simulink model "sf_electrohydraulic"  (Simulink 7.6)
settings: Solver=ode45  SolverMode=SingleTasking  StartTime=0.0  StopTime=2  FixedStep=0.2e-4  RelTol=1e-6
model workspace (MAT data in the model file):
  BHcurve.H = [-11439.2615347; -7246.13776302; -3771.53605391; -987.067511384; -118.29393547; -78.4550283852; -44.7231237731; -17.3583519401; -13.039382708; -10.5700097302; -8.52378165855; -6.82818955541; -5.42314941344; -4.25887305422; -3.43177169131; -2.84371281009; -2.35642206816; -1.95263211657; -1.61803449144; -1.34077258756; -1.11102151473; -0.920639948664; -0.762881639861; -0.632156357415; -0.523831796886; -0.434069432681; -0.359688498308; -0.298053274602; -0.246979691925; -0.204657936755; -0.1695883202; -0.140528135894; -0.116447624191; -0.0964934822022; -0.0799586266544; -0.0662571381046; -0.0549034986404; -0.0454953873528; -0.0376994239281; -0.0312393551788; -0.0258862658976; -0.0214504671522; -0.01777477458; -0.0147289384949; -0.0122050284356; -0.0101136086056; -0.00838056867855; -0.00694449766789; -0.0057545078036; -0.00476843130279; 0; 0.00476843130279; 0.0057545078036; 0.00694449766789; 0.00838056867855; 0.0101136086056; 0.0122050284356; 0.0147289384949; 0.01777477458; 0.0214504671522; 0.0258862658976; 0.0312393551788; 0.0376994239281; 0.0454953873528; 0.0549034986404; 0.0662571381046; 0.0799586266544; 0.0964934822022; 0.116447624191; 0.140528135894; 0.1695883202; 0.204657936755; 0.246979691925; 0.298053274602; 0.359688498308; 0.434069432681; 0.523831796886; 0.632156357415; 0.762881639861; 0.920639948664; 1.11102151473; 1.34077258756; 1.61803449144; 1.95263211657; 2.35642206816; 2.84371281009; 3.43177169131; 4.25887305422; 5.42314941344; 6.82818955541; 8.52378165855; 10.5700097302; 13.039382708; 16.3583519401; 43.7231237731; 77.4550283852; 118.29393547; 987.067511384; 3771.53605391; 7246.13776302; 11439.2615347]
  BHcurve.B = [-3; -2.48592831856; -2.05994653501; -1.70695980871; -1.41445990904; -1.17208198112; -0.971237262845; -0.804808738584; -0.666898944758; -0.552620990798; -0.457925390153; -0.379456565057; -0.314433940246; -0.260553412125; -0.2159057019; -0.178908699498; -0.14825140084; -0.122847451871; -0.101796653157; -0.0843530609392; -0.0698985543155; -0.0579209318665; -0.0479957615882; -0.0397713409677; -0.0329562342596; -0.0273089453397; -0.0226293601901; -0.0187516557758; -0.0155384240377; -0.0128758027804; -0.0106694409187; -0.00884115510766; -0.00732615928365; -0.00607076894318; -0.00503049881043; -0.00416848648312; -0.00345418619798; -0.00286228642905; -0.00237181296327; -0.00196538567058; -0.0016286026318; -0.00134952980069; -0.00111827811609; -0.000926653078943; -0.00076786437681; -0.000636285266376; -0.000527253187456; -0.00043690454325; -0.000362037792192; -0.0003; 0; 0.0003; 0.000362037792192; 0.00043690454325; 0.000527253187456; 0.000636285266376; 0.00076786437681; 0.000926653078943; 0.00111827811609; 0.00134952980069; 0.0016286026318; 0.00196538567058; 0.00237181296327; 0.00286228642905; 0.00345418619798; 0.00416848648312; 0.00503049881043; 0.00607076894318; 0.00732615928365; 0.00884115510766; 0.0106694409187; 0.0128758027804; 0.0155384240377; 0.0187516557758; 0.0226293601901; 0.0273089453397; 0.0329562342596; 0.0397713409677; 0.0479957615882; 0.0579209318665; 0.0698985543155; 0.0843530609392; 0.101796653157; 0.122847451871; 0.14825140084; 0.178908699498; 0.2159057019; 0.260553412125; 0.314433940246; 0.379456565057; 0.457925390153; 0.552620990798; 0.666898944758; 0.804808738584; 0.971237262845; 1.17208198112; 1.41445990904; 1.70695980871; 2.05994653501; 2.48592831856; 3]
  BHcurve.Hn = [-11439.2615347 -7246.13776302 -3771.53605391 -987.067511384 -118.29393547 -79 -45 -18 -13.9460730484 -12.2551666032 -10.8540091978 -9.69295024023 -8.73084712615 -7.93360733394 -7.27298034189 -6.72555655937 -6.2719377983 -5.89604989031 -5.58457309194 -5.32647009407 -5.11259491023 -4.93536878485 -4.78851163689 -4.66681952259 -4.56598023156 -4.48242048183 -4.41317929912 -4.35580309348 -4.30825871534 -4.26886141001 -4.23621511767 -4.20916300347 -4.18674646454 -4.16817116157 -4.15277887101 -4.14002416068 -4.12945506214 -4.12069705502 -4.11343979572 -4.10742612025 -4.10244293153 -4.09831364821 -4.09489194743 -4.09205657981 -4.08970707293 -4.08776017103 -4.08614688483 -4.08481004689 -4.08370228579 -4.08278434756 -4.07834541673 -4.07324748496 -4.07219327019 -4.07092105156 -4.06938574748 -4.06753295381 -4.06529701606 -4.06259870282 -4.05934239827 -4.05541271391 -4.05067039973 -4.04494740989 -4.03804094786 -4.02970628032 -4.01964806486 -4.00750988447 -3.9928616177 -3.97518419717 -3.95385121616 -3.92810673168 -3.89703847727 -3.8595455365 -3.81429933149 -3.75969654427 -3.6938023025 -3.61428161647 -3.51831663779 -3.40250680776 -3.26274835716 -3.09408888752 -2.89055188078 -2.64492491894 -2.34850410906 -1.99078565716 -1.55909366199 -1.03813093919 -0.409436959267 0.584138774493 2.11545170072 3.9634288706 6.19355411929 8.88485285711 12.1326923677 16 43 77 118.29393547 987.067511384 3771.53605391 7246.13776302 11439.2615347]
  BHcurve.Hp : numeric (value not decoded)
PreLoadFcn:
  | sf_electrohydraulic_data
values from neighbouring files (symbols this model uses):
  A = sort(A)    [emldemo_uniquetol.m]    (also in sf_electrohydraulic_data.m = 8e-05)
  Ao = 2.58064e-006    (= 2.58064e-06)    [sf_electrohydraulic_data.m]
  Ap = 0.0005    [sf_electrohydraulic_data.m]
  beta = 1.5004e+009    (= 1500400000)    [sf_electrohydraulic_data.m]
  Cv = 8.48528    [sf_electrohydraulic_data.m]
  dcmax = 85    [sf_electrohydraulic_data.m]
  dcmin = 10    [sf_electrohydraulic_data.m]
  deltai = 0.1    [sf_electrohydraulic_data.m]
  Fs0 = 2    [sf_electrohydraulic_data.m]
  gmax = 0.001016    [sf_electrohydraulic_data.m]
  gser = 0.0001905    [sf_electrohydraulic_data.m]
  Ihold = 1    [sf_electrohydraulic_data.m]
  Ipull = 2.5    [sf_electrohydraulic_data.m]
  Ka = 38000    [sf_electrohydraulic_data.m]
  Ki = 253080    [sf_electrohydraulic_data.m]
  Ko = 0.0307568    [sf_electrohydraulic_data.m]
  Ks = 8998.88    [sf_electrohydraulic_data.m]
  Ksp = 17322.8    [sf_electrohydraulic_data.m]
  Lsteel = 0.05    [sf_electrohydraulic_data.m]
  m = s.find('-regexp','name','eml_asteroids')    [eml_asteroids_setup.m]    (also in sf_edit_icon.m = sz(1); sf_electrohydraulic_data.m = 0.001)
  Mp = 1    [sf_electrohydraulic_data.m]
  mu0 = 1.25664e-006    (= 1.25664e-06)    [sf_electrohydraulic_data.m]
  N = 200    [sf_electrohydraulic_data.m]    (also in sf_pool_plotter.m = size(p,1))
  Ps = 682001    [sf_electrohydraulic_data.m]
  R = 2    [sf_electrohydraulic_data.m]
  Tpwm = 0.02    [sf_electrohydraulic_data.m]
  Vd = 0.5    [sf_electrohydraulic_data.m]
  Vs = 14    [sf_electrohydraulic_data.m]
  Vz = 50    [sf_electrohydraulic_data.m]
undefined symbols (not defined in the file or in its folder): Newton, Raphson
libraries: simulink x2
settings Model: Creator=The MathWorks Inc.  CovMetricSettings=dcmtr  ExtModeTrigMode=oneshot  ExtModeArmWhenConnect=off  ExtModeAutoUpdateStatusClock=off
settings SolverCC: ShapePreserveControl=EnableAll
settings DataIOCC: LimitDataPoints=off  SaveFormat=StructureWithTime
settings OptimizationCC: BooleanDataType=off  InlineInvariantSignals=on  InitFltsAndDblsToZero=on
settings DebuggingCC: SaveWithParameterizedLinksMsg=none  SignalResolutionControl=TryResolveAllWithWarning  SolverPrmCheckMsg=none  MultiTaskDSMMsg=warning  MultiTaskCondExecSysMsg=none  IntegerOverflowMsg=none  StrictBusMsg=None
settings HardwareCC: TargetUnknown=on
settings SFSimCC: SimCustomHeaderCode=#include <math.h>  SimParseCustomCode=off
settings RTWCC: IncludeERTFirstTime=on
settings GRTTargetCC: TargetFcnLib=ansi_tfl_tmw.mat

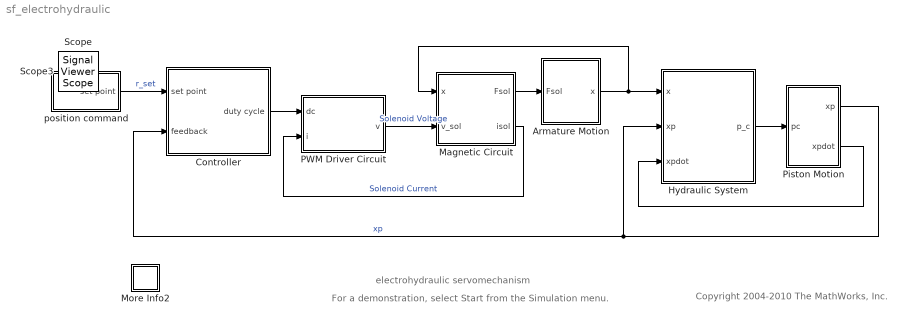
== system sf_electrohydraulic ==
  note: electrohydraulic servomechanism
  note: For a demonstration, select Start from the Simulation menu.
  note: Copyright 2004-2010 The MathWorks, Inc.
  Armature Motion : Subsystem
  Controller : Subsystem
  Hydraulic System : Subsystem
  Magnetic Circuit : Subsystem
  More Info2 : Subsystem
      settings: OpenFcn=showdemo(bdroot(gcs))
      mask Display: disp('?')
  PWM Driver Circuit : Stateflow chart  TreatAsAtomicUnit=on
  Piston Motion : Subsystem
  position command : Subsystem
  Scope : SignalViewerScope  IOType=viewer  RefreshTime=0.035000
      settings: TimeRange=0.02  YMin=-0.25  YMax=2.75
  Scope3 : SignalViewerScope  IOType=viewer  RefreshTime=0.035000
      settings: ShowLegends=on  TimeRange=2  YMin=0.002  YMax=0.018  SaveName=ScopeData3
  wires:
  position command/1(set point) -> Controller/1(set point)  "r_set"
  Piston Motion/2(xpdot) -> Hydraulic System/3(xpdot)
  Piston Motion/1(xp) -> Hydraulic System/2(xp), Controller/2(feedback)  "xp"
  Armature Motion/1(x) -> Magnetic Circuit/1(x), Hydraulic System/1(x)
  Controller/1(duty cycle) -> PWM Driver Circuit/1(dc)
  PWM Driver Circuit/1(v) -> Magnetic Circuit/2(v_sol)  "Solenoid Voltage"
  Magnetic Circuit/1(Fsol) -> Armature Motion/1(Fsol)
  Magnetic Circuit/2(isol) -> PWM Driver Circuit/2(i)  "Solenoid Current"
  Hydraulic System/1(p_c) -> Piston Motion/1(pc)

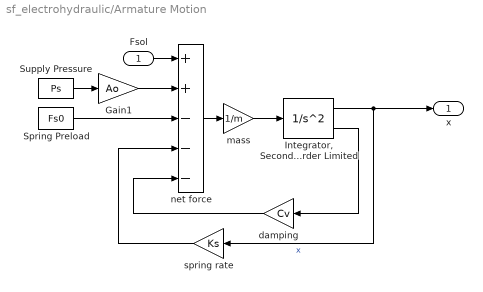
== system sf_electrohydraulic/Armature Motion ==
  Fsol : Inport
  Gain1 : Gain  Gain=Ao  SaturateOnIntegerOverflow=on  OutDataTypeStr=Inherit: Same as input  ParamDataTypeStr=Inherit: Same as input
  "Integrator, Second-Order Limited" : SecondOrderIntegrator  LimitX=on  UpperLimitX=gmax - gmin  LowerLimitX=0  ReinitDXDTwhenXreachesSaturation=on
  Spring Preload : Constant  Value=Fs0
  Supply Pressure : Constant  Value=Ps
  damping : Gain  Gain=Cv  SaturateOnIntegerOverflow=on  OutDataTypeStr=Inherit: Same as input  ParamDataTypeStr=Inherit: Same as input
  mass : Gain  Gain=1/m  SaturateOnIntegerOverflow=on  OutDataTypeStr=Inherit: Same as input  ParamDataTypeStr=Inherit: Same as input
  net force : Sum  Inputs=++---  SaturateOnIntegerOverflow=on  InputSameDT=on  OutDataTypeStr=Inherit: Same as first input
  spring rate : Gain  Gain=Ks  SaturateOnIntegerOverflow=on  OutDataTypeStr=Inherit: Same as input  ParamDataTypeStr=Inherit: Same as input
  x : Outport
  wires:
  mass/1 -> "Integrator, Second-Order Limited"/1
  Fsol/1 -> net force/1
  spring rate/1 -> net force/4
  Spring Preload/1 -> net force/3
  damping/1 -> net force/5
  "Integrator, Second-Order Limited"/2 -> damping/1
  net force/1 -> mass/1
  "Integrator, Second-Order Limited"/1 -> x/1, spring rate/1  "x"
  Gain1/1 -> net force/2
  Supply Pressure/1 -> Gain1/1

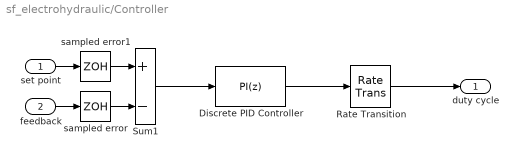
== system sf_electrohydraulic/Controller ==
  set point : Inport
  feedback : Inport  Port=2
  Discrete PID Controller : simulink/Continuous/PID Controller  DialogController=pidpack.PIDConfig.pidDDGCreate  DialogControllerArgs=DataTag1  SystemSampleTime=-1  Controller=PI  TimeDomain=Discrete-time  SampleTime=Tpwm  IntegratorMethod=Forward Euler  FilterMethod=Forward Euler  Form=Parallel  P=Ka  I=Ki  D=0  N=100  InitialConditionSource=internal  InitialConditionForIntegrator=dcnull  InitialConditionForFilter=0  ExternalReset=none  LimitOutput=on  UpperSaturationLimit=dcmax  LowerSaturationLimit=dcmin  LinearizeAsGain=off  AntiWindupMode=clamping  Kb=1  TrackingMode=off  Kt=1  PParamMin=[]  PParamMax=[]  IParamMin=[]  IParamMax=[]  DParamMin=[]  DParamMax=[]  NParamMin=[]  NParamMax=[]  KbParamMin=[]  KbParamMax=[]  KtParamMin=[]  KtParamMax=[]  POutMin=[]  POutMax=[]  IOutMin=[]  IOutMax=[]  DOutMin=[]  DOutMax=[]  NOutMin=[]  NOutMax=[]  KbOutMin=[]  KbOutMax=[]  KtOutMin=[]  KtOutMax=[]  IntegratorOutMin=[]  IntegratorOutMax=[]  FilterOutMin=[]  FilterOutMax=[]  SumOutMin=[]  SumOutMax=[]  SumI1OutMin=[]  SumI1OutMax=[]  SumI2OutMin=[]  SumI2OutMax=[]  SumI3OutMin=[]  SumI3OutMax=[]  SumDOutMin=[]  SumDOutMax=[]  SaturationOutMin=[]  SaturationOutMax=[]  IntegratorContinuousStateAttributes=''  IntegratorStateMustResolveToSignalObject=off  IntegratorRTWStateStorageClass=Auto  FilterContinuousStateAttributes=''  FilterStateMustResolveToSignalObject=off  FilterRTWStateStorageClass=Auto
  Rate Transition : RateTransition  Integrity=off
  Sum1 : Sum  Inputs=+-  SaturateOnIntegerOverflow=on  InputSameDT=on  OutDataTypeStr=Inherit: Same as first input
  sampled error : ZeroOrderHold  SampleTime=Tpwm
  sampled error1 : ZeroOrderHold  SampleTime=Tpwm
  duty cycle : Outport
  wires:
  Sum1/1 -> Discrete PID Controller/1
  set point/1 -> sampled error1/1
  feedback/1 -> sampled error/1
  Discrete PID Controller/1 -> Rate Transition/1
  sampled error/1 -> Sum1/2
  sampled error1/1 -> Sum1/1
  Rate Transition/1 -> duty cycle/1

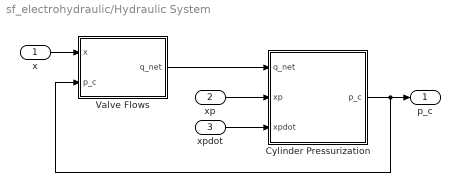
== system sf_electrohydraulic/Hydraulic System ==
  x : Inport
  xp : Inport  Port=2
  xpdot : Inport  Port=3
  Cylinder Pressurization : Subsystem
  Valve Flows : Subsystem
  p_c : Outport
  wires:
  Valve Flows/1(q_net) -> Cylinder Pressurization/1(q_net)
  Cylinder Pressurization/1(p_c) -> p_c/1, Valve Flows/2(p_c)
  x/1 -> Valve Flows/1(x)
  xp/1 -> Cylinder Pressurization/2(xp)
  xpdot/1 -> Cylinder Pressurization/3(xpdot)

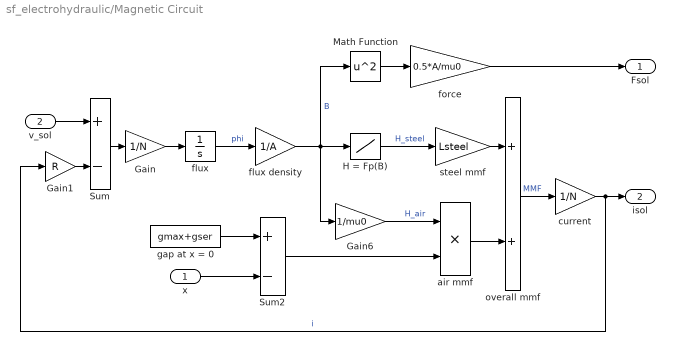
== system sf_electrohydraulic/Magnetic Circuit ==
  x : Inport
  v_sol : Inport  Port=2
  Gain : Gain  Gain=1/N  SaturateOnIntegerOverflow=on  OutDataTypeStr=Inherit: Same as input  ParamDataTypeStr=Inherit: Same as input
  Gain1 : Gain  Gain=R  SaturateOnIntegerOverflow=on  OutDataTypeStr=Inherit: Same as input  ParamDataTypeStr=Inherit: Same as input
  Gain6 : Gain  Gain=1/mu0  SaturateOnIntegerOverflow=on  OutDataTypeStr=Inherit: Same as input  ParamDataTypeStr=Inherit: Same as input
  H = Fp(B) : Lookup  InputValues=BHcurve.B  Table=0.5*(BHcurve.Hp+BHcurve.Hn)
  Math Function : Math  Operator=square  SaturateOnIntegerOverflow=on
  Sum : Sum  Inputs=+-  SaturateOnIntegerOverflow=on  InputSameDT=on  OutDataTypeStr=Inherit: Same as first input
  Sum2 : Sum  Inputs=+-  SaturateOnIntegerOverflow=on  InputSameDT=on  OutDataTypeStr=Inherit: Same as first input
  air mmf : Product  SaturateOnIntegerOverflow=on  RndMeth=Zero  InputSameDT=on  OutDataTypeStr=Inherit: Same as first input
  current : Gain  Gain=1/N  SaturateOnIntegerOverflow=on  OutDataTypeStr=Inherit: Same as input  ParamDataTypeStr=Inherit: Same as input
  flux : Integrator  LowerSaturationLimit=0
  flux density : Gain  Gain=1/A  SaturateOnIntegerOverflow=on  OutDataTypeStr=Inherit: Same as input  ParamDataTypeStr=Inherit: Same as input
  force : Gain  Gain=0.5*A/mu0  SaturateOnIntegerOverflow=on  OutDataTypeStr=Inherit: Same as input  ParamDataTypeStr=Inherit: Same as input
  gap at x = 0 : Constant  Value=gmax+gser
  overall mmf : Sum  SaturateOnIntegerOverflow=on  InputSameDT=on  OutDataTypeStr=Inherit: Same as first input
  steel mmf : Gain  Gain=Lsteel  SaturateOnIntegerOverflow=on  OutDataTypeStr=Inherit: Same as input  ParamDataTypeStr=Inherit: Same as input
  Fsol : Outport
  isol : Outport  Port=2
  wires:
  x/1 -> Sum2/2
  gap at x = 0/1 -> Sum2/1
  Sum2/1 -> air mmf/2
  Sum/1 -> Gain/1
  Gain1/1 -> Sum/2
  v_sol/1 -> Sum/1
  current/1 -> isol/1, Gain1/1  "i"
  flux density/1 -> H = Fp(B)/1, Math Function/1, Gain6/1  "B"
  overall mmf/1 -> current/1  "MMF"
  air mmf/1 -> overall mmf/2
  steel mmf/1 -> overall mmf/1
  H = Fp(B)/1 -> steel mmf/1  "H_steel"
  Gain6/1 -> air mmf/1  "H_air"
  Gain/1 -> flux/1
  flux/1 -> flux density/1  "phi"
  force/1 -> Fsol/1
  Math Function/1 -> force/1

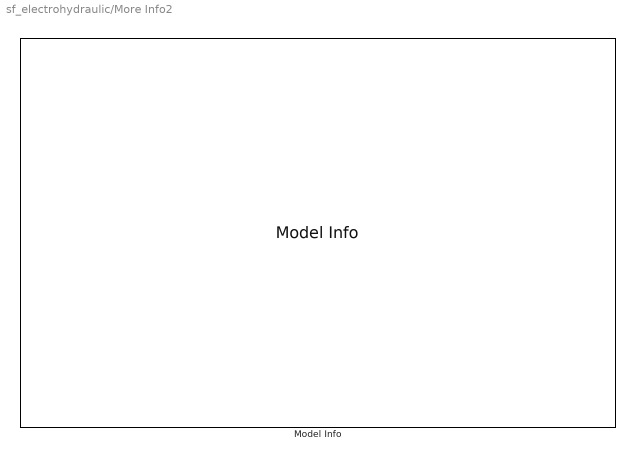
== system sf_electrohydraulic/More Info2 ==
  Model Info : simulink/Model-Wide Utilities/Model Info  SystemSampleTime=-1  InitialBlockCM=none  BlockCM=None  Frame=on  DisplayStringWithTags=Model Info  HorizontalTextAlignment=Left  LeftAlignmentValue=0.02  SourceBlockDiagram=sf_electrohydraulic  TagMaxNumber=20

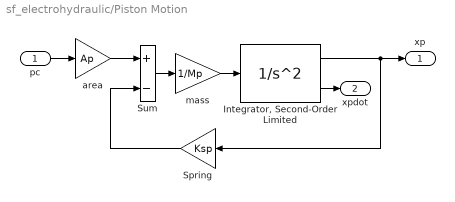
== system sf_electrohydraulic/Piston Motion ==
  pc : Inport
  "Integrator, Second-Order Limited" : SecondOrderIntegrator  ICX=xpmin  LimitX=on  UpperLimitX=xpmax  LowerLimitX=xpmin  StateNameX='PistonPosition'  StateNameDXDT='PistonVelocity'  ReinitDXDTwhenXreachesSaturation=on
  Spring : Gain  Gain=Ksp  SaturateOnIntegerOverflow=on  OutDataTypeStr=Inherit: Same as input  ParamDataTypeStr=Inherit: Same as input
  Sum : Sum  Inputs=+-  SaturateOnIntegerOverflow=on  InputSameDT=on  OutDataTypeStr=Inherit: Same as first input
  area : Gain  Gain=Ap  SaturateOnIntegerOverflow=on  OutDataTypeStr=Inherit: Same as input  ParamDataTypeStr=Inherit: Same as input
  mass : Gain  Gain=1/Mp  SaturateOnIntegerOverflow=on  OutDataTypeStr=Inherit: Same as input  ParamDataTypeStr=Inherit: Same as input
  xp : Outport
  xpdot : Outport  Port=2
  wires:
  pc/1 -> area/1
  "Integrator, Second-Order Limited"/2 -> xpdot/1
  area/1 -> Sum/1
  Sum/1 -> mass/1
  Spring/1 -> Sum/2
  mass/1 -> "Integrator, Second-Order Limited"/1
  "Integrator, Second-Order Limited"/1 -> xp/1, Spring/1

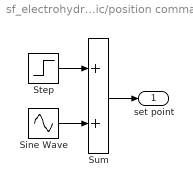
== system sf_electrohydraulic/position command ==
  Sine Wave : Sin  Amplitude=2e-3  Frequency=3*2*pi  SampleTime=0
  Step : Step  Before=0.01  After=0.015  SampleTime=0
  Sum : Sum  SaturateOnIntegerOverflow=on  InputSameDT=on  OutDataTypeStr=Inherit: Same as first input
  set point : Outport
  wires:
  Step/1 -> Sum/1
  Sine Wave/1 -> Sum/2
  Sum/1 -> set point/1

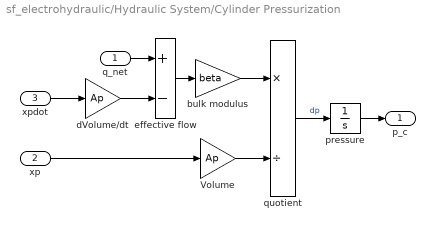
== system sf_electrohydraulic/Hydraulic System/Cylinder Pressurization ==
  q_net : Inport
  xp : Inport  Port=2
  xpdot : Inport  Port=3
  Volume : Gain  Gain=Ap  SaturateOnIntegerOverflow=on  OutDataTypeStr=Inherit: Same as input  ParamDataTypeStr=Inherit: Same as input
  bulk modulus : Gain  Gain=beta  SaturateOnIntegerOverflow=on  OutDataTypeStr=Inherit: Same as input  ParamDataTypeStr=Inherit: Same as input
  dVolume/dt : Gain  Gain=Ap  SaturateOnIntegerOverflow=on  OutDataTypeStr=Inherit: Same as input  ParamDataTypeStr=Inherit: Same as input
  effective flow : Sum  Inputs=+-  SaturateOnIntegerOverflow=on  InputSameDT=on  OutDataTypeStr=Inherit: Same as first input
  pressure : Integrator  LimitOutput=on  LowerSaturationLimit=0
  quotient : Product  Inputs=*/  SaturateOnIntegerOverflow=on  RndMeth=Zero  InputSameDT=on  OutDataTypeStr=Inherit: Same as first input
  p_c : Outport
  wires:
  dVolume/dt/1 -> effective flow/2
  bulk modulus/1 -> quotient/1
  quotient/1 -> pressure/1  "dp"
  effective flow/1 -> bulk modulus/1
  xp/1 -> Volume/1
  Volume/1 -> quotient/2
  xpdot/1 -> dVolume/dt/1
  q_net/1 -> effective flow/1
  pressure/1 -> p_c/1

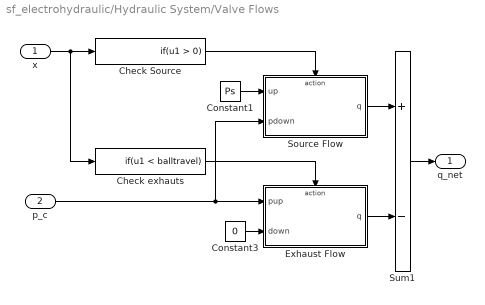
== system sf_electrohydraulic/Hydraulic System/Valve Flows ==
  x : Inport
  p_c : Inport  Port=2
  Check Source : If  ShowElse=off
  Check exhauts : If  IfExpression=u1 < balltravel  ShowElse=off
  Constant1 : Constant  Value=Ps
  Constant3 : Constant  Value=0
  Exhaust Flow : Subsystem  mask(turbulent orifice flow){Ko=Ko, Ao=Ao}
      mask prompts: Ko "flow coefficient"; Ao "orifice area"
      mask Display: plot(-0.75,-1.25,0.75,1.25,[0 0],[1 -1],0.5*cos(-pi/4:.1:pi/4)-0.55, 0.5*sin(-pi/4:.1:pi/4),-0.5*cos(-pi/4:.1:pi/4)+0.55, 0.5*sin(-pi/4:.1:pi/4))
  Source Flow : Subsystem  mask(turbulent orifice flow){Ko=Ko, Ao=Ao}
      mask prompts: Ko "flow coefficient"; Ao "orifice area"
      mask Display: plot(-0.75,-1.25,0.75,1.25,[0 0],[1 -1],0.5*cos(-pi/4:.1:pi/4)-0.55, 0.5*sin(-pi/4:.1:pi/4),-0.5*cos(-pi/4:.1:pi/4)+0.55, 0.5*sin(-pi/4:.1:pi/4))
  Sum1 : Sum  Inputs=+-  SaturateOnIntegerOverflow=on  InputSameDT=on  OutDataTypeStr=Inherit: Same as first input
  q_net : Outport
  wires:
  x/1 -> Check Source/1, Check exhauts/1
  Check Source/1 -> Source Flow/Action
  Exhaust Flow/1(q) -> Sum1/2
  Source Flow/1(q) -> Sum1/1
  Constant3/1 -> Exhaust Flow/2(down)
  Constant1/1 -> Source Flow/1(up)
  Check exhauts/1 -> Exhaust Flow/Action
  p_c/1 -> Exhaust Flow/1(pup), Source Flow/2(pdown)
  Sum1/1 -> q_net/1

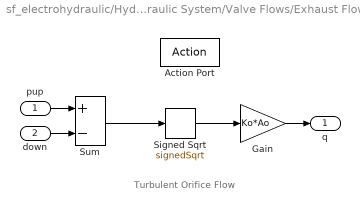
== system sf_electrohydraulic/Hydraulic System/Valve Flows/Exhaust Flow ==
  note: Turbulent Orifice Flow
  pup : Inport
  down : Inport  Port=2
  Action Port : ActionPort  ActionType=then
  Gain : Gain  Gain=Ko*Ao  SaturateOnIntegerOverflow=on  OutDataTypeStr=Inherit: Same as input  ParamDataTypeStr=Inherit: Same as input
  Signed Sqrt : Sqrt  Operator=signedSqrt  AlgorithmType=Newton-Raphson  SaturateOnIntegerOverflow=on
  Sum : Sum  Inputs=+-  SaturateOnIntegerOverflow=on  InputSameDT=on  OutDataTypeStr=Inherit: Same as first input
  q : Outport  OutputWhenDisabled=reset  InitialOutput=0
  wires:
  down/1 -> Sum/2
  Sum/1 -> Signed Sqrt/1
  Signed Sqrt/1 -> Gain/1
  pup/1 -> Sum/1
  Gain/1 -> q/1

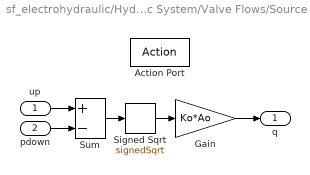
== system sf_electrohydraulic/Hydraulic System/Valve Flows/Source Flow ==
  up : Inport
  pdown : Inport  Port=2
  Action Port : ActionPort  ActionType=then
  Gain : Gain  Gain=Ko*Ao  SaturateOnIntegerOverflow=on  OutDataTypeStr=Inherit: Same as input  ParamDataTypeStr=Inherit: Same as input
  Signed Sqrt : Sqrt  Operator=signedSqrt  AlgorithmType=Newton-Raphson  SaturateOnIntegerOverflow=on
  Sum : Sum  Inputs=+-  SaturateOnIntegerOverflow=on  InputSameDT=on  OutDataTypeStr=Inherit: Same as first input
  q : Outport  OutputWhenDisabled=reset  InitialOutput=0
  wires:
  Sum/1 -> Signed Sqrt/1
  Gain/1 -> q/1
  pdown/1 -> Sum/2
  up/1 -> Sum/1
  Signed Sqrt/1 -> Gain/1

== stateflow chart PWM Driver Circuit ==
  settings: updateMethod=CONTINUOUS
  settings: description=|
      | The objective is to direct fluid from supply to control when the duty
      |  cycle is high, and from control to exhaust when low.  The solenoid
      | is energized for the high portion.  This requires a current which is
      | initially large to pull the solenoid armature into its energized position,
      | and then somewhat lower to hold it in for the remainder of the high
      | phase of each PWM pulse.
  state Main [parallel]
    settings: executionOrder=1
    state ON
      state pull_in_current
        entry : v = Vs;
      state regulate_hold_current
        state freewheel
          entry: v = -Vd;
        state hold/
          entry : v = Vs;
        (default) -> freewheel
        freewheel -> hold : [ i <= Ihold - deltai ]
        hold -> freewheel : [ i >= Ihold + deltai ]
      (default) -> pull_in_current
      pull_in_current -> regulate_hold_current : [ i >= Ipull ]
    state OFF
      state Discharge_Solenoid
        entry : v = -Vz;
      state Solenoid_OFF
        entry : v = 0;
      Discharge_Solenoid -> Solenoid_OFF : [i < 0]
      (default) -> Discharge_Solenoid
    (default) -> (junction 12)
    (junction 12) -> ON : { toff = ton + dc*Tpwm/100; }
    OFF -> (junction 12) : [ t >= ton ]
    ON -> OFF : [ t > toff ]
        | { ton += Tpwm;}
  data: v output double; dc input double [0..100]; ton local double; toff local double; Tpwm parameter double; Ipull parameter double; Ihold parameter double; deltai parameter double; Vs parameter double; Vz parameter double; Vd parameter double; i input double
  data v settings: description=applied solenoid voltage
  data dc settings: description=pulse-width modulation duty cycle
  data ton settings: description=absolute time at the beginning of each PWM cycle
  data toff settings: description=absolute time at which the current PWM cycle switches off
  data Tpwm settings: description=pulse-width modulation period
  data Ipull settings: description=solenoid pull-in current, generates maximum force to move armature
  data Ihold settings: description=solenoid hold current (maintain armature in energized position)
  data deltai settings: description=switch-mode current regulation error width
  data Vs settings: description=power supply voltage
  data Vz settings: description=zener diode voltage
  data Vd settings: description=freewheel diode forward voltage drop
  data i settings: description=solenoid current
